simulink model "BebeEnvioIP"  (R2020a)
settings: Solver=FixedStepAuto  StartTime=0.0  StopTime=10.0  RelTol=1e-3
undefined symbols (not defined in the file): frec_cardiaca, untitled1, ventilacion
libraries: androidcommunicationlib x3, androiduilib x3, simulink x1, visionsources x1, androidaudiovideolib x1
settings Model: Creator=luisi  LastModifiedBy=luisi
settings OptimizationCC: EnhancedBackFolding=on  PassReuseOutputArgsAs=Individual arguments  ZeroExternalMemoryAtStartup=off  ZeroInternalMemoryAtStartup=off  MaxStackSize=64  OptimizeBlockOrder=speed  DifferentSizesBufferReuse=on  OptimizationCustomize=off  EfficientTunableParamExpr=on
settings DebuggingCC: ParameterTunabilityLossMsg=error
settings HardwareCC: ProdBitPerPointer=32  ProdBitPerSizeT=32  ProdBitPerPtrDiffT=32  ProdLargestAtomicInteger=Long  ProdLargestAtomicFloat=Double  ProdWordSize=32  ProdHWDeviceType=ARM Compatible->ARM Cortex
settings SFSimCC: MATLABDynamicMemAlloc=off
settings RTWCC: SystemTargetFile=ert.tlc  HardwareBoard=Android Device  TemplateMakefile=ert_default_tmf  RTWVerbose=off  Toolchain=Android SDK/NDK Tools
settings CodeAppCC: ForceParamTrailComments=on  IgnoreCustomStorageClasses=off  OperatorAnnotations=on  SimulinkDataObjDesc=on  SFDataObjDesc=on  InsertBlockDesc=on
settings ERTTargetCC: ExtModeMexArgs='192.168.0.180'

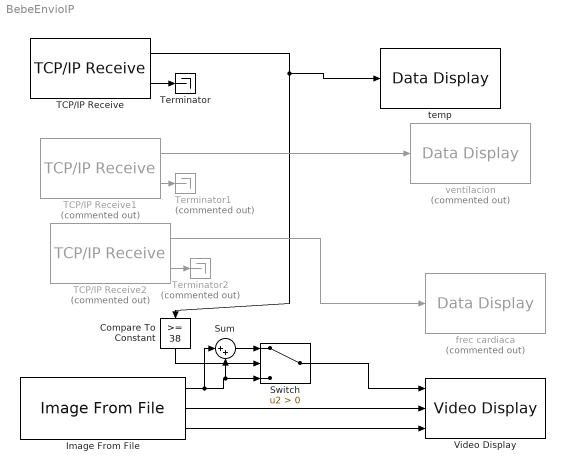
== system BebeEnvioIP ==
  Compare To Constant : simulink/Logic and Bit Operations/Compare To Constant  relop=>=  const=38  OutDataTypeStr=boolean
  Image From File : visionsources/Image From File  Tag=vipblks_nd  FileName=C:\Users\luisi\Downloads\victoria.jpg  Ts=inf  imagePorts=Separate color signals  OutPortLabels=R|G|B  ImageDataType=uint8  sdImageDataType=uint(8)  Signed=on  WordLength=16  FractionLengthMode=User-defined  FractionLength=15
  Sum : Sum  Inputs=|++
  Switch : Switch  Criteria=u2 > Threshold
  TCP/IP Receive : androidcommunicationlib/TCP//IP Receive  TCPReceiveId=BebeEnvioIP/TCP//IP_Receive  Mode_=Client  LocalServerPort_=25000  RemoteAddr_=192.168.0.149  RemoteServerPort_=25002  DataType_=uint8  DataSize_=1  SampleTime_=0.1  SimulateUsing=Code generation  ClientPortBindingSelection_=off  ClientPortToBind_=35000  BlockingMode_=off  BlockTimeout_=0.1
      settings: SourceProductBaseCode=ANDROID
  TCP/IP Receive1 : androidcommunicationlib/TCP//IP Receive  Commented=on  TCPReceiveId=untitled1/TCP//IP_Receive1  Mode_=Client  LocalServerPort_=25000  RemoteAddr_=192.168.0.149  RemoteServerPort_=25001  DataType_=uint8  DataSize_=1  SampleTime_=0.1  SimulateUsing=Code generation  ClientPortBindingSelection_=off  ClientPortToBind_=35000  BlockingMode_=off  BlockTimeout_=0.1
      settings: SourceProductBaseCode=ANDROID
  TCP/IP Receive2 : androidcommunicationlib/TCP//IP Receive  Commented=on  TCPReceiveId=untitled1/TCP//IP_Receive2  Mode_=Client  LocalServerPort_=25000  RemoteAddr_=192.168.0.149  RemoteServerPort_=25000  DataType_=uint8  DataSize_=1  SampleTime_=0.1  SimulateUsing=Code generation  ClientPortBindingSelection_=off  ClientPortToBind_=35000  BlockingMode_=off  BlockTimeout_=0.1
      settings: SourceProductBaseCode=ANDROID
  Terminator : Terminator
  Terminator1 : Terminator  Commented=on
  Terminator2 : Terminator  Commented=on
  Video Display : androidaudiovideolib/Video Display  BlockPlatform=Android
      settings: SourceProductBaseCode=ANDROID
  frec cardiaca : androiduilib/Data Display  Commented=on  DataDisplayId=untitled1/frec_cardiaca  Format=Integer  Precision=6  SimulateUsing=Code generation  blockPlatform=Android
      settings: SourceProductBaseCode=ANDROID
  temp : androiduilib/Data Display  DataDisplayId=BebeEnvioIP/temp  Format=Float  Precision=2  SimulateUsing=Code generation  blockPlatform=Android
      settings: SourceProductBaseCode=ANDROID
  ventilacion : androiduilib/Data Display  Commented=on  DataDisplayId=untitled1/ventilacion  Format=Integer  Precision=6  SimulateUsing=Code generation  blockPlatform=Android
      settings: SourceProductBaseCode=ANDROID
  wires:
  TCP/IP Receive/1 -> Compare To Constant/1, temp/1
  Sum/1 -> Switch/1
  Compare To Constant/1 -> Switch/2
  TCP/IP Receive2/1 -> frec cardiaca/1
  Image From File/1 -> Sum/1, Sum/2, Switch/3
  Image From File/3 -> Video Display/3
  Image From File/2 -> Video Display/2
  TCP/IP Receive1/1 -> ventilacion/1
  Switch/1 -> Video Display/1
  TCP/IP Receive/2 -> Terminator/1
  TCP/IP Receive1/2 -> Terminator1/1
  TCP/IP Receive2/2 -> Terminator2/1
